simulink model "natural_balloon"  (R2013a)
settings: Solver=ode45  StartTime=0.0  StopTime=s_dash_end  RelTol=1e-3
undefined symbols (not defined in the file): a_dash, epsilon, k, m0, r0, rho, S0, tb, theta_0, V0, z0
settings Model: Creator=Willdog  LastModifiedBy=Willdog
settings DebuggingCC: SolverPrmCheckMsg=none

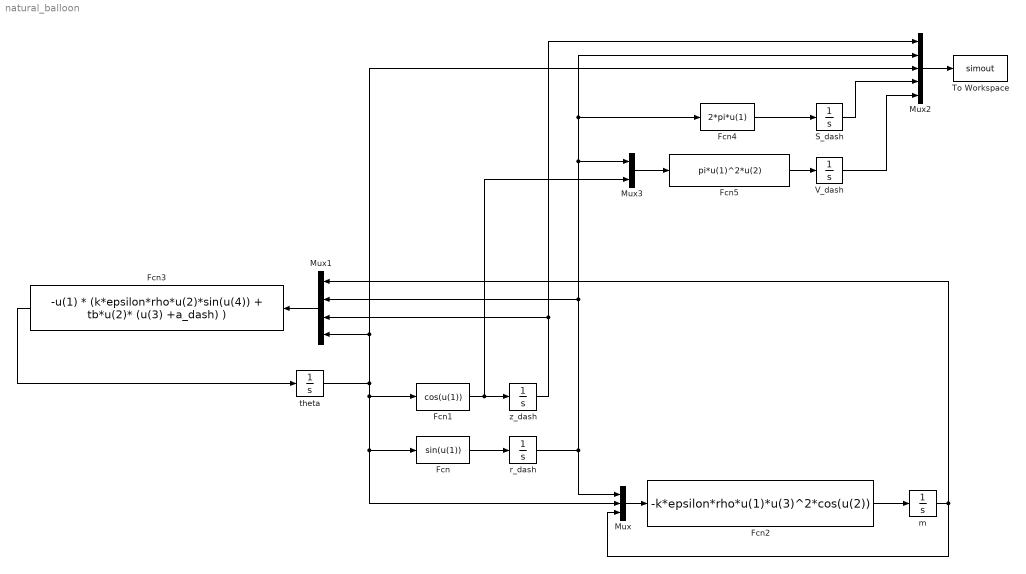
== system natural_balloon ==
  Fcn : Fcn  Expr=sin(u(1))
  Fcn1 : Fcn  Expr=cos(u(1))
  Fcn2 : Fcn  Expr=-k*epsilon*rho*u(1)*u(3)^2*cos(u(2))
  Fcn3 : Fcn  Expr=-u(1) * (k*epsilon*rho*u(2)*sin(u(4)) + tb*u(2)* (u(3) +a_dash) )
  Fcn4 : Fcn  Expr=2*pi*u(1)
  Fcn5 : Fcn  Expr=pi*u(1)^2*u(2)
  Mux : Mux  Inputs=3
  Mux1 : Mux
  Mux2 : Mux  Inputs=5
  Mux3 : Mux  Inputs=2
  S_dash : Integrator  InitialCondition=S0
  To Workspace : ToWorkspace  VariableName=simout  SampleTime=-1  SaveFormat=Timeseries
  V_dash : Integrator  InitialCondition=V0
  m : Integrator  InitialCondition=m0
  r_dash : Integrator  InitialCondition=r0
  theta : Integrator  InitialCondition=theta_0
  z_dash : Integrator  InitialCondition=z0
  wires:
  theta/1 -> Mux2/3, Mux1/4, Fcn/1, Mux/2, Fcn1/1
  Fcn/1 -> r_dash/1
  Fcn1/1 -> Mux3/2, z_dash/1
  r_dash/1 -> Mux/1, Mux3/1, Fcn4/1, Mux2/2, Mux1/2
  Fcn2/1 -> m/1
  m/1 -> Mux/3, Mux1/1
  Mux/1 -> Fcn2/1
  z_dash/1 -> Mux2/1, Mux1/3
  Mux1/1 -> Fcn3/1
  Fcn3/1 -> theta/1
  Mux2/1 -> To Workspace/1
  S_dash/1 -> Mux2/4
  V_dash/1 -> Mux2/5
  Fcn4/1 -> S_dash/1
  Mux3/1 -> Fcn5/1
  Fcn5/1 -> V_dash/1
